simulink model "create_index_vector_test"  (R2020b)
settings: Solver=FixedStepDiscrete  StartTime=0.0  StopTime=10.0  FixedStep=0.1  RelTol=1e-3
undefined symbols (not defined in the file): kContainerIndexVector
libraries: create_index_vector_lib x1
settings Model: Creator=rsub  LastModifiedBy=rsub

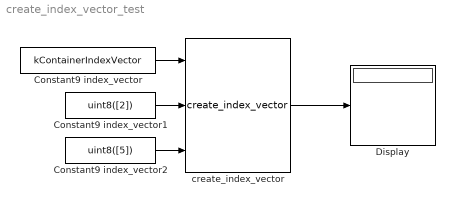
== system create_index_vector_test ==
  Constant9 index_vector : Constant  Value=kContainerIndexVector
  Constant9 index_vector1 : Constant  Value=uint8([2])
  Constant9 index_vector2 : Constant  Value=uint8([5])
  Display : Display
  create_index_vector : create_index_vector_lib/create_index_vector  vector_length=kContainerLength
  wires:
  Constant9 index_vector/1 -> create_index_vector/1
  Constant9 index_vector1/1 -> create_index_vector/2
  Constant9 index_vector2/1 -> create_index_vector/3
  create_index_vector/1 -> Display/1
